simulink model "foward_simple"  (R2023b)
settings: Solver=VariableStepAuto  StartTime=0.0  StopTime=12  RelTol=1e-3
values from neighbouring files (symbols this model uses):
  A = 1.4    [forward_sim_data.m]
  Cd = 0.7    [forward_sim_data.m]
  drive = 1    [forward_sim_data.m]
  eff = 0.9    [forward_sim_data.m]
  f = 0.015    [forward_sim_data.m]
  g = 9.81    [forward_sim_data.m]
  hca = .25    (= 0.25)    [forward_sim_data.m]
  k = 0.6    [forward_sim_data.m]
  L = 3.05    [forward_sim_data.m]
  LDR = -3.3    [forward_sim_data.m]
  m = 620    [forward_sim_data.m]
  mu = 2.25    [forward_sim_data.m]
  P = 745*745    (= 555025)    [forward_sim_data.m]
  rho = 1.2    [forward_sim_data.m]
settings Model: Creator=jc2fb  LastModifiedBy=Pat
settings DataIOCC: ReturnWorkspaceOutputs=off

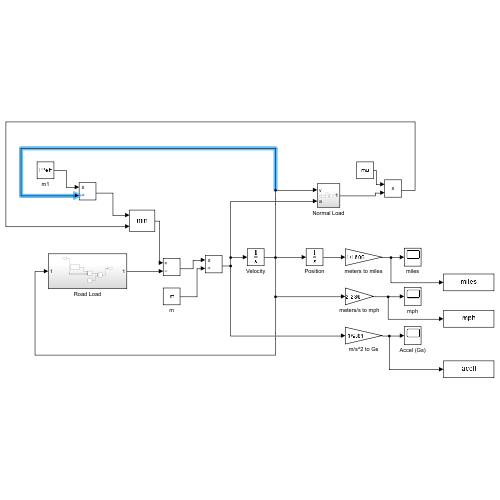
[thumbnail: Simulink's stored preview of the top-level diagram]
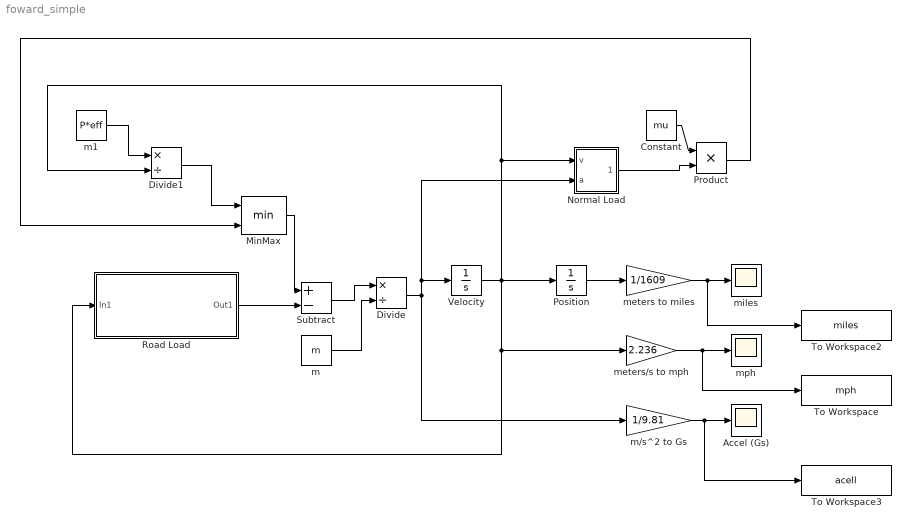
== system foward_simple ==
  Accel (Gs) : Scope
  Constant : Constant  Value=mu
  Divide : Product  Inputs=*/
  Divide1 : Product  Inputs=*/
  MinMax : MinMax  Inputs=2
  Normal Load : Subsystem
  Position : Integrator
  Product : Product
  Road Load : Subsystem
  Subtract : Sum  Inputs=+-
  To Workspace : ToWorkspace  VariableName=mph  SampleTime=-1
  To Workspace2 : ToWorkspace  VariableName=miles  SampleTime=-1
  To Workspace3 : ToWorkspace  VariableName=acell  SampleTime=-1
  Velocity : Integrator  InitialCondition=0.01
  m : Constant  Value=m  VectorParams1D=off
  m/s^2 to Gs : Gain  Gain=1/9.81
  m1 : Constant  Value=P*eff  VectorParams1D=off
  meters to miles : Gain  Gain=1/1609
  meters/s to mph : Gain  Gain=2.236
  miles : Scope
  mph : Scope
  wires:
  meters to miles/1 -> To Workspace2/1, miles/1
  Position/1 -> meters to miles/1
  meters/s to mph/1 -> To Workspace/1, mph/1
  Velocity/1 -> Road Load/1(In1), meters/s to mph/1, Normal Load/1(v), Divide1/2, Position/1
  m/s^2 to Gs/1 -> To Workspace3/1, Accel (Gs)/1
  Divide/1 -> Normal Load/2(a), Velocity/1, m/s^2 to Gs/1
  MinMax/1 -> Subtract/1
  Subtract/1 -> Divide/1
  m/1 -> Divide/2
  Road Load/1(Out1) -> Subtract/2
  Product/1 -> MinMax/2
  Constant/1 -> Product/1
  Normal Load/1(Out1) -> Product/2
  m1/1 -> Divide1/1
  Divide1/1 -> MinMax/1

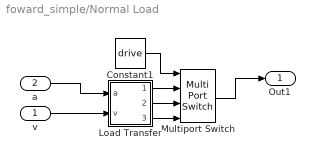
== system foward_simple/Normal Load ==
  v : Inport
  a : Inport  Port=2
  Constant1 : Constant  Value=drive
  Load Transfer : Subsystem
  Multiport Switch : MultiPortSwitch  SaturateOnIntegerOverflow=off  InputSameDT=off
  Out1 : Outport
  wires:
  Constant1/1 -> Multiport Switch/1
  Load Transfer/3(AWD) -> Multiport Switch/4
  Load Transfer/2(FWD) -> Multiport Switch/3
  Multiport Switch/1 -> Out1/1
  Load Transfer/1(RWD) -> Multiport Switch/2
  a/1 -> Load Transfer/1(a)
  v/1 -> Load Transfer/2(v)

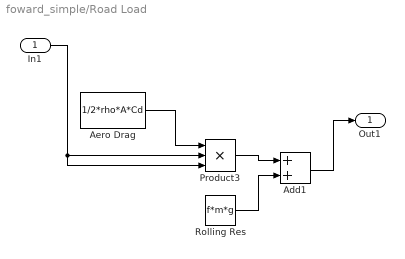
== system foward_simple/Road Load ==
  In1 : Inport
  Add1 : Sum
  Aero Drag : Constant  Value=1/2*rho*A*Cd
  Product3 : Product  Inputs=3
  Rolling Res : Constant  Value=f*m*g
  Out1 : Outport
  wires:
  Aero Drag/1 -> Product3/1
  Rolling Res/1 -> Add1/2
  Add1/1 -> Out1/1
  In1/1 -> Product3/3, Product3/2
  Product3/1 -> Add1/1

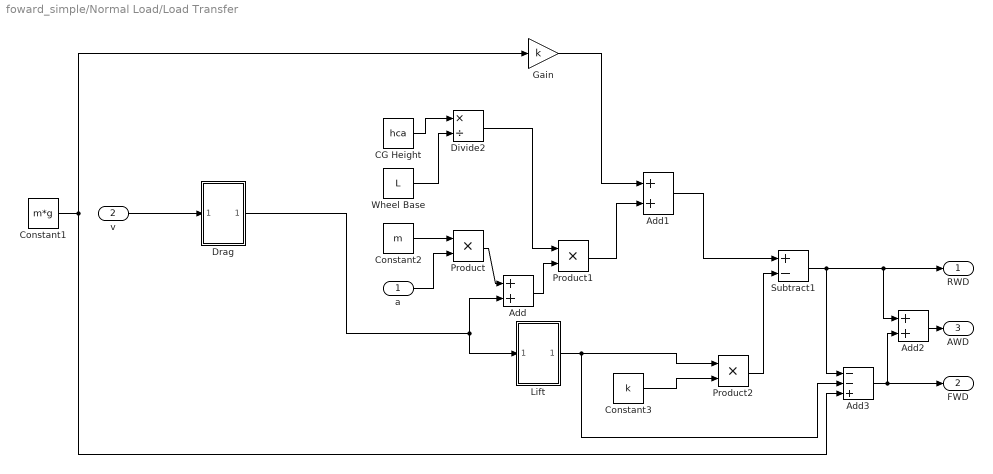
== system foward_simple/Normal Load/Load Transfer ==
  a : Inport
  v : Inport  Port=2
  Add : Sum
  Add1 : Sum
  Add2 : Sum
  Add3 : Sum  Inputs=--+
  CG Height : Constant  Value=hca
  Constant1 : Constant  Value=m*g
  Constant2 : Constant  Value=m
  Constant3 : Constant  Value=k
  Divide2 : Product  Inputs=*/
  Drag : Subsystem
  Gain : Gain  Gain=k
  Lift : Subsystem
  Product : Product
  Product1 : Product
  Product2 : Product
  Subtract1 : Sum  Inputs=+-
  Wheel Base : Constant  Value=L
  RWD : Outport
  FWD : Outport  Port=2
  AWD : Outport  Port=3
  wires:
  Product2/1 -> Subtract1/2
  Constant3/1 -> Product2/2
  Wheel Base/1 -> Divide2/2
  CG Height/1 -> Divide2/1
  Divide2/1 -> Product1/1
  Add1/1 -> Subtract1/1
  Constant2/1 -> Product/1
  Add/1 -> Product1/2
  Product1/1 -> Add1/2
  Subtract1/1 -> Add3/1, Add2/1, RWD/1
  Product/1 -> Add/1
  a/1 -> Product/2
  Drag/1(Out1) -> Lift/1(In1), Add/2
  v/1 -> Drag/1(In1)
  Lift/1(Out1) -> Add3/2, Product2/1
  Constant1/1 -> Gain/1, Add3/3
  Gain/1 -> Add1/1
  Add3/1 -> Add2/2, FWD/1
  Add2/1 -> AWD/1

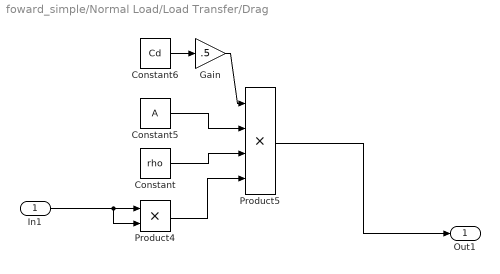
== system foward_simple/Normal Load/Load Transfer/Drag ==
  In1 : Inport
  Constant : Constant  Value=rho
  Constant5 : Constant  Value=A
  Constant6 : Constant  Value=Cd
  Gain : Gain  Gain=.5
  Product4 : Product
  Product5 : Product  Inputs=4
  Out1 : Outport
  wires:
  In1/1 -> Product4/2, Product4/1
  Constant6/1 -> Gain/1
  Constant/1 -> Product5/3
  Product4/1 -> Product5/4
  Constant5/1 -> Product5/2
  Product5/1 -> Out1/1
  Gain/1 -> Product5/1

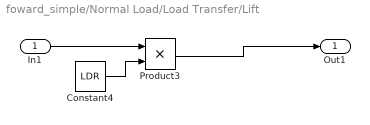
== system foward_simple/Normal Load/Load Transfer/Lift ==
  In1 : Inport
  Constant4 : Constant  Value=LDR
  Product3 : Product
  Out1 : Outport
  wires:
  Constant4/1 -> Product3/2
  In1/1 -> Product3/1
  Product3/1 -> Out1/1
